simulink model "led_res"  (R2026a)
settings: Solver=VariableStepAuto  StopTime=200e-9  MaxStep=1e-10
values from neighbouring files (symbols this model uses):
  HT_0 = (h * c / (lambda * q)) * eta_int * eta_inj * eta_ext    [LEDcbV2.m]    (also in led_mask_init.m = ((h * c) / (lambda * q)) * eta_int * eta_inj * eta_ext)
Description:
  | Author: Puspendu Rana
  | Project: LED Simulation
  | Date: April 2026
settings Model: Creator=Puspendu Rana  LastModifiedBy=HP

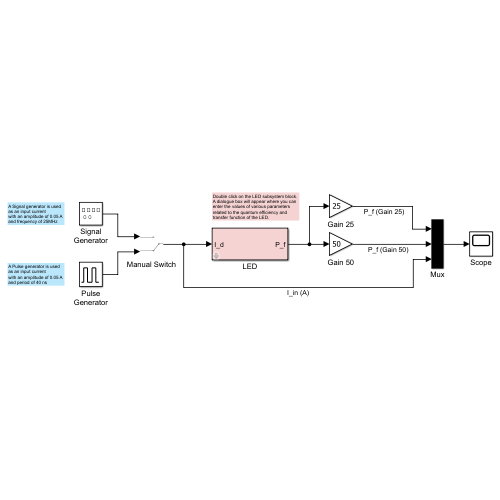
[thumbnail: Simulink's stored preview of the top-level diagram]
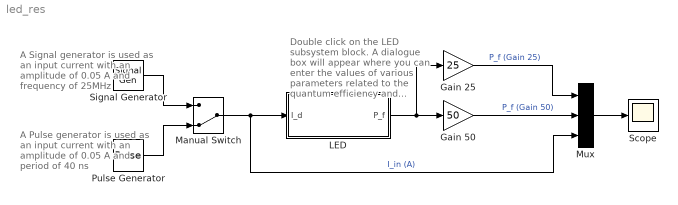
== system led_res ==
  note: Double click on the LED subsystem block.
      | A dialogue box will appear where you can
      | enter the values of various parameters
      | related to the quantum efficiency and
      | transfer function of the LED.
  note: A Pulse generator is used
      | as an input current
      | with an amplitude of 0.05 A
      | and period of 40 ns
  note: A Signal generator is used
      | as an input current
      | with an amplitude of 0.05 A
      | and frequency of 25MHz
  Gain 25 : Gain  Gain=25
  Gain 50 : Gain  Gain=50
  LED : Subsystem  mask{lambda=1310, tau_r=2.5, tau_nr=10, eta_inj=1, n_s=3.62, n_a=1}
      mask prompts: lambda "Emission wavelength (nm)"; tau_r "Radiative recombination time (ns)"; tau_nr "Nonradiative recombination time (ns)"; eta_inj "Current-injection efficiency"; n_s "Semiconductor refraction index"; n_a "Media refraction index (Air=1)"
  Manual Switch : ManualSwitch  CurrentSetting=0
  Mux : Mux  Inputs=3
  Pulse Generator : DiscretePulseGenerator  PulseType=Time based  Amplitude=0.05  Period=40e-9  PulseWidth=50
  Scope : Scope
      settings: Title=Response of an LED  ActiveDisplayYMinimum=-0.0062499999999999986  ActiveDisplayYMaximum=0.05625  YLabel=Amplitude
  Signal Generator : SignalGenerator  WaveForm=square  Amplitude=0.05  Frequency=25e6
  wires:
  LED/1(P_f) -> Gain 50/1, Gain 25/1
  Gain 50/1 -> Mux/2  "P_f (Gain 50)"
  Mux/1 -> Scope/1
  Gain 25/1 -> Mux/1  "P_f (Gain 25)"
  Signal Generator/1 -> Manual Switch/1
  Pulse Generator/1 -> Manual Switch/2
  Manual Switch/1 -> Mux/3, LED/1(I_d)  "I_in (A)"

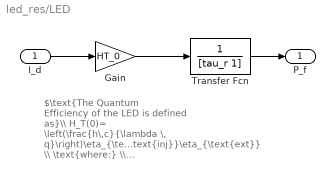
== system led_res/LED ==
  note: $\text{The Quantum Efficiency of the LED is defined as}\\ H_T(0)= \left(\frac{h\,c}{\lambda \, q}\right)\eta_{\text{int}}\eta_{\text{inj}}\eta_{\text{ext}} \\ \text{where:} \\ \eta_{\text{int}} = \frac{\tau_{\text{nr}}}{\tau_{\text{nr}} + \tau_{\text{r}}}\\ \eta_{ext} = \left[1 - \left(\frac{n_s - n_m}{n_s + n_m}\right)^2\right]\left[1 - \text{cos}\left(\frac{n_m}{n_s}\right)\right]$
  I_d : Inport
  "Gain " : Gain  Gain=HT_0
  Transfer Fcn : TransferFcn  Denominator=[tau_r 1]
  P_f : Outport
  wires:
  Transfer Fcn/1 -> P_f/1
  I_d/1 -> "Gain "/1
  "Gain "/1 -> Transfer Fcn/1
